simulink model "TRABALHO"  (R2021b)
settings: Solver=VariableStepAuto  StartTime=0.0  StopTime=10.0  RelTol=1e-3
libraries: simulink x1
settings Model: Creator=gusta  LastModifiedBy=gusta

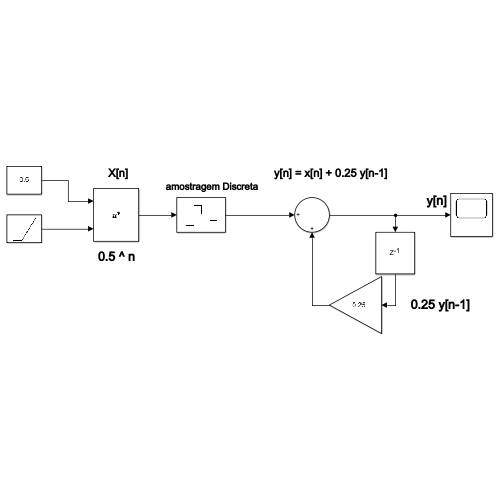
[thumbnail: Simulink's stored preview of the top-level diagram]
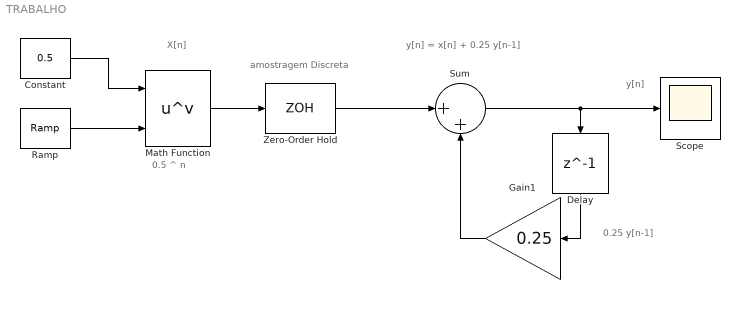
== system TRABALHO ==
  note: 0.5 ^ n
  note: y[n] = x[n] + 0.25 y[n-1]
  note: amostragem Discreta
  note: 0.25 y[n-1]
  note: y[n]
  note: X[n]
  Constant : Constant  Value=0.5
  Delay : Delay  DelayLength=1  InitialCondition=8
  Gain1 : Gain  Gain=0.25
  Math Function : Math  Operator=pow  OutputSignalType=real  SaturateOnIntegerOverflow=on
  Ramp : simulink/Sources/Ramp  slope=1  start=0  InitialOutput=0
  Scope : Scope
  Sum : Sum  Inputs=|++
  Zero-Order Hold : ZeroOrderHold
  wires:
  Sum/1 -> Scope/1, Delay/1
  Delay/1 -> Gain1/1
  Gain1/1 -> Sum/2
  Constant/1 -> Math Function/1
  Ramp/1 -> Math Function/2
  Zero-Order Hold/1 -> Sum/1
  Math Function/1 -> Zero-Order Hold/1
